simulink model "unresponsive_nonterminating"  (R2015a)
settings: Solver=ode45  StartTime=0.0  StopTime=10.0  RelTol=1e-3
libraries: simulink x9
settings Model: Creator=shafiul  LastModifiedBy=shafiul

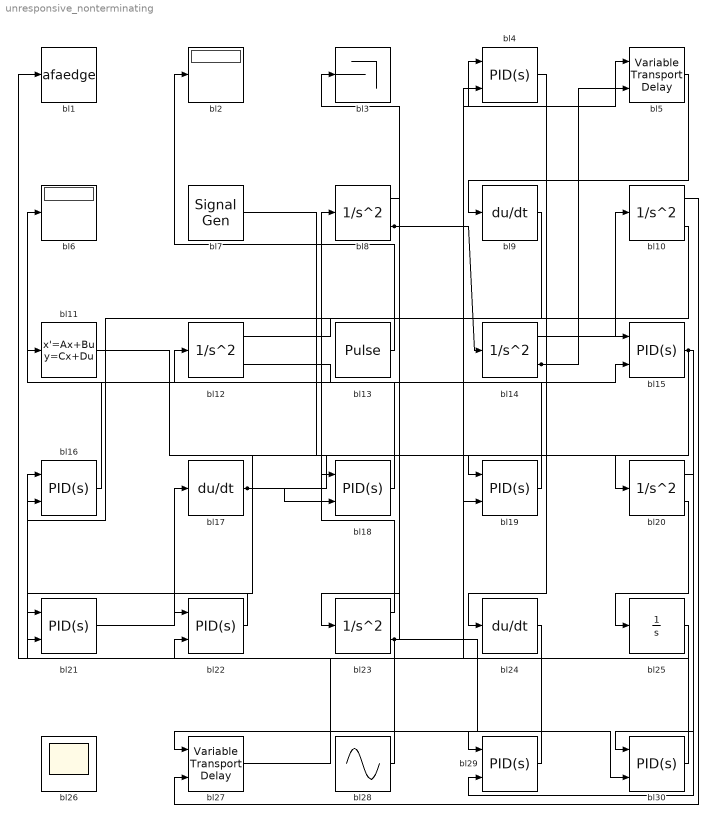
== system unresponsive_nonterminating ==
  bl1 : ToWorkspace  VariableName=afaedge  SaveFormat=Timeseries  SampleTime=-1
  bl{8,10,12,14,20,23} (6 alike) : SecondOrderIntegrator
  bl11 : StateSpace  X0=0
  bl13 : DiscretePulseGenerator  PulseType=Time based  Period=10  PulseWidth=5
  bl{4,15,18..19,21..22,29..30} (8 alike) : simulink/Continuous/PID Controller (2DOF)  Controller=PID  TimeDomain=Continuous-time  SampleTime=-1  IntegratorMethod=Forward Euler  FilterMethod=Forward Euler  Form=Parallel  UseFilter=on  ControllerParametersSource=internal  P=1  I=1  D=0  N=100  b=1  c=1  InitialConditionSource=internal  InitialConditionForIntegrator=0  InitialConditionForFilter=0  ExternalReset=none  LimitOutput=off  UpperSaturationLimit=inf  LowerSaturationLimit=-inf  LinearizeAsGain=on  AntiWindupMode=none  Kb=1  TrackingMode=off  Kt=1  PParamMin=[]  PParamMax=[]  IParamMin=[]  IParamMax=[]  DParamMin=[]  DParamMax=[]  NParamMin=[]  NParamMax=[]  bParamMin=[]  bParamMax=[]  cParamMin=[]  cParamMax=[]  KbParamMin=[]  KbParamMax=[]  KtParamMin=[]  KtParamMax=[]  POutMin=[]  POutMax=[]  IOutMin=[]  IOutMax=[]  DOutMin=[]  DOutMax=[]  NOutMin=[]  NOutMax=[]  bOutMin=[]  bOutMax=[]  cOutMin=[]  cOutMax=[]  KbOutMin=[]  KbOutMax=[]  KtOutMin=[]  KtOutMax=[]  IntegratorOutMin=[]  IntegratorOutMax=[]  FilterOutMin=[]  FilterOutMax=[]  SumOutMin=[]  SumOutMax=[]  Sum1OutMin=[]  Sum1OutMax=[]  Sum2OutMin=[]  Sum2OutMax=[]  Sum3OutMin=[]  Sum3OutMax=[]  SumI1OutMin=[]  SumI1OutMax=[]  SumI2OutMin=[]  SumI2OutMax=[]  SumI3OutMin=[]  SumI3OutMax=[]  SumDOutMin=[]  SumDOutMax=[]  SaturationOutMin=[]  SaturationOutMax=[]  IntegratorContinuousStateAttributes=''  IntegratorStateMustResolveToSignalObject=off  IntegratorRTWStateStorageClass=Auto  FilterContinuousStateAttributes=''  FilterStateMustResolveToSignalObject=off  FilterRTWStateStorageClass=Auto  DifferentiatorICPrevScaledInput=0  DifferentiatorOutMin=[]  DifferentiatorOutMax=[]
  bl16 : simulink/Continuous/PID Controller (2DOF)  Controller=PID  TimeDomain=Continuous-time  SampleTime=-1  IntegratorMethod=Forward Euler  FilterMethod=Forward Euler  Form=Parallel  UseFilter=on  ControllerParametersSource=internal  P=1  I=1  D=0  N=100  b=1  c=1  InitialConditionSource=internal  InitialConditionForIntegrator=1  InitialConditionForFilter=2  ExternalReset=none  LimitOutput=off  UpperSaturationLimit=inf  LowerSaturationLimit=-inf  LinearizeAsGain=on  AntiWindupMode=none  Kb=1  TrackingMode=off  Kt=1  PParamMin=[]  PParamMax=[]  IParamMin=[]  IParamMax=[]  DParamMin=[]  DParamMax=[]  NParamMin=[]  NParamMax=[]  bParamMin=[]  bParamMax=[]  cParamMin=[]  cParamMax=[]  KbParamMin=[]  KbParamMax=[]  KtParamMin=[]  KtParamMax=[]  POutMin=[]  POutMax=[]  IOutMin=[]  IOutMax=[]  DOutMin=[]  DOutMax=[]  NOutMin=[]  NOutMax=[]  bOutMin=[]  bOutMax=[]  cOutMin=[]  cOutMax=[]  KbOutMin=[]  KbOutMax=[]  KtOutMin=[]  KtOutMax=[]  IntegratorOutMin=[]  IntegratorOutMax=[]  FilterOutMin=[]  FilterOutMax=[]  SumOutMin=[]  SumOutMax=[]  Sum1OutMin=[]  Sum1OutMax=[]  Sum2OutMin=[]  Sum2OutMax=[]  Sum3OutMin=[]  Sum3OutMax=[]  SumI1OutMin=[]  SumI1OutMax=[]  SumI2OutMin=[]  SumI2OutMax=[]  SumI3OutMin=[]  SumI3OutMax=[]  SumDOutMin=[]  SumDOutMax=[]  SaturationOutMin=[]  SaturationOutMax=[]  IntegratorContinuousStateAttributes=''  IntegratorStateMustResolveToSignalObject=off  IntegratorRTWStateStorageClass=Auto  FilterContinuousStateAttributes=''  FilterStateMustResolveToSignalObject=off  FilterRTWStateStorageClass=Auto  DifferentiatorICPrevScaledInput=0  DifferentiatorOutMin=[]  DifferentiatorOutMax=[]
  bl17 : Derivative
  bl2 : Display
  bl24 : Derivative
  bl25 : Integrator
  bl26 : Scope
      settings: Floating=on
  bl27 : VariableTransportDelay  MaximumDelay=10  InitialOutput=2
  bl28 : Sin  SampleTime=0
  bl3 : Terminator
  bl5 : VariableTransportDelay  MaximumDelay=10  InitialOutput=1
  bl6 : Display
  bl7 : SignalGenerator  Units=rad/sec
  bl9 : Derivative
  wires:
  bl29/1 -> bl27/1
  bl16/1 -> bl6/1
  bl18/1 -> bl12/1
  bl5/1 -> bl9/1
  bl9/1 -> bl16/1
  bl30/1 -> bl1/1
  bl28/1 -> bl16/2
  bl4/1 -> bl24/1
  bl22/1 -> bl21/1
  bl17/1 -> bl20/1, bl18/2
  bl23/1 -> bl8/1
  bl14/1 -> bl10/1
  bl24/1 -> bl29/1
  bl12/1 -> bl15/1
  bl25/1 -> bl21/2
  bl15/1 -> bl29/2, bl22/1
  bl23/2 -> bl11/1, bl30/2, bl22/2
  bl21/1 -> bl17/1
  bl13/1 -> bl2/1
  bl8/1 -> bl23/1
  bl8/2 -> bl14/1, bl5/1
  bl12/2 -> bl15/2
  bl7/1 -> bl19/1
  bl11/1 -> bl19/2
  bl14/2 -> bl4/1, bl5/2
  bl27/1 -> bl4/2
  bl20/1 -> bl30/1
  bl10/1 -> bl27/2
  bl10/2 -> bl18/1
  bl19/1 -> bl3/1
  bl20/2 -> bl25/1
